simulink subsystem "PitchSubsystem"  (R2023b)
settings: Solver=VariableStepAuto  StartTime=0.0  StopTime=10.0  RelTol=1e-3
values from neighbouring files (symbols this model uses):
  Ixx = 15.67*10^(-3)    (= 0.01567)    [drone_input_params.m]
  Iyy = 15.67*10^(-3)    (= 0.01567)    [drone_input_params.m]
  Izz = 28.346*10^(-3)    (= 0.028346)    [drone_input_params.m]
  Jr = 6.01*10^(-5)    (= 6.01e-05)    [drone_input_params.m]
  l = 0.3    [drone_input_params.m]
settings Model: Creator=FRESH  LastModifiedBy=FRESH

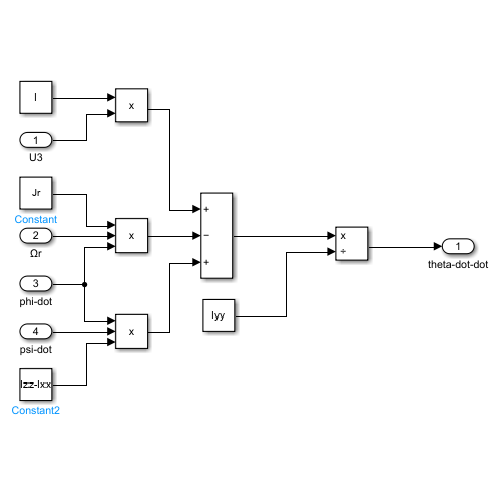
[thumbnail: Simulink's stored preview of the top-level diagram]
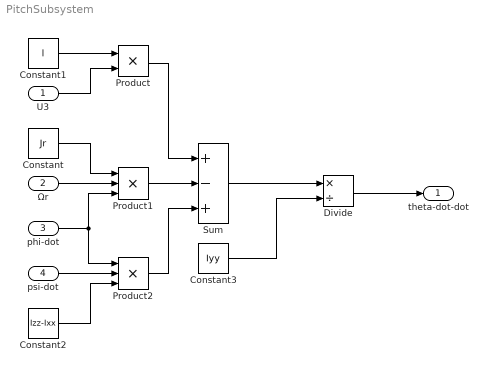
== system PitchSubsystem ==
  U3 : Inport
  Ωr : Inport  Port=2
  phi-dot : Inport  Port=3
  psi-dot : Inport  Port=4
  Constant : Constant  Value=Jr
  Constant1 : Constant  Value=l
  Constant2 : Constant  Value=Izz-Ixx
  Constant3 : Constant  Value=Iyy
  Divide : Product  Inputs=*/
  Product : Product
  Product1 : Product  Inputs=3
  Product2 : Product  Inputs=3
  Sum : Sum  Inputs=+-+
  theta-dot-dot : Outport
  wires:
  Constant2/1 -> Product2/3
  Constant1/1 -> Product/1
  U3/1 -> Product/2
  Constant/1 -> Product1/1
  Ωr/1 -> Product1/2
  Product/1 -> Sum/1
  phi-dot/1 -> Product2/1, Product1/3
  psi-dot/1 -> Product2/2
  Product1/1 -> Sum/2
  Product2/1 -> Sum/3
  Sum/1 -> Divide/1
  Constant3/1 -> Divide/2
  Divide/1 -> theta-dot-dot/1
